simulink model "bandwidth_admittance"  (R2020b)
settings: Solver=ode4  StartTime=0.0  StopTime=5  FixedStep=1e-5  MaxStep=1e-4  RelTol=1e-4  EnableMultiTasking=on
values from neighbouring files (symbols this model uses):
  Be = 2 * sqrt(Ke * Je)    [bandwidth.m]    (also in bandwidth_reference.m = 2 * sqrt(Ke * 0.0001))
  D = 0.1    [bandwidth.m]    (also in bandwidth_reference.m = 0.9; frequency_max_modulation_force.m = 0.9; frequency_max_modulation_force_sea.m = 0.9; frequency_max_modulation_position.m = 0.9)
  dm = 0.0068    [bandwidth.m]    (also in bandwidth_reference.m; frequency_max_modulation_force.m; frequency_max_modulation_force_sea.m; frequency_max_modulation_position.m)
  gear = 103    [bandwidth_reference.m]    (also in frequency_max_position.m; frequency_max_velocity.m; frequency_position.m; frequency_velocity.m)
  Jm = 0.0064    [bandwidth.m]    (also in bandwidth_reference.m = 0.0104; frequency_max_modulation_force.m = 0.0104; frequency_max_modulation_force_sea.m = 0.0104; frequency_max_modulation_position.m = 0.0104)
  Ke = 1e-2    (= 0.01)    [bandwidth.m]    (also in bandwidth_reference.m = 20)
  kt = 1.5038    [bandwidth_reference.m]    (also in frequency_max_modulation_force.m; frequency_max_modulation_force_sea.m; frequency_max_modulation_position.m; frequency_max_modulation_velocity.m)
  P = 15    [bandwidth.m]    (also in bandwidth_reference.m = 1; frequency_max_modulation_force.m = 10; frequency_max_modulation_force_sea.m = 10; frequency_max_modulation_position.m = 10)
  qe = 0    [bandwidth.m]    (also in bandwidth_reference.m)
settings Model: Creator=eldisondimo  LastModifiedBy=filippo
settings DataIOCC: LimitDataPoints=on  SaveOutput=off  SaveTime=off  ReturnWorkspaceOutputs=off
settings OptimizationCC: ExpressionDepthLimit=2147483647  LifeSpan=1
settings DebuggingCC: UnderspecifiedInitializationDetection=Classic  MergeDetectMultiDrivingBlocksExec=none  FcnCallInpInsideContextMsg=warning  AllowSymbolicDim=off  StateNameClashWarn=warning  SFUnexpectedBacktrackingDiag=warning  SFNoUnconditionalDefaultTransitionDiag=warning  SFExecutionAtInitializationDiag=none  ArithmeticOperatorsInVariantConditions=warning
settings SFSimCC: SimUseLocalCustomCode=off  CustomCodeUndefinedFunction=UseInterfaceOnly
settings RTWCC: RTWUseLocalCustomCode=off
settings CodeAppCC: StateflowObjectComments=on
settings GRTTargetCC: TargetLangStandard=C89/C90 (ANSI)  CombineOutputUpdateFcns=off  GRTInterface=on

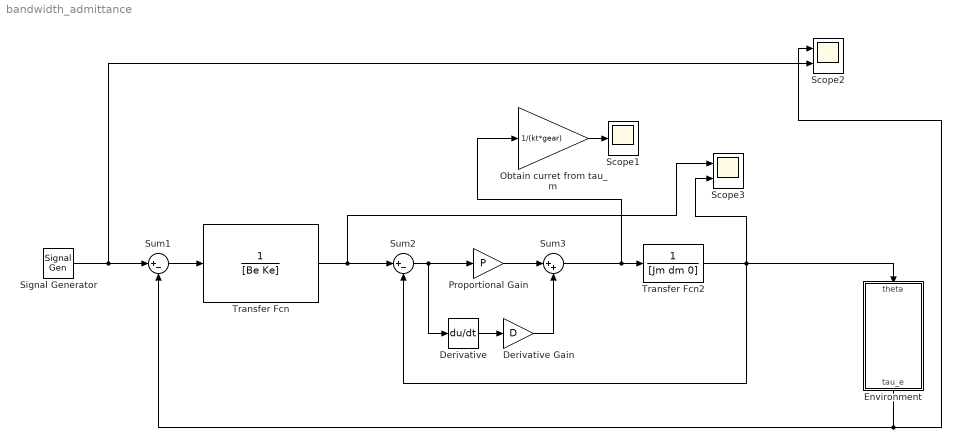
== system bandwidth_admittance ==
  Derivative : Derivative
  Derivative Gain : Gain  Gain=D
  Environment : Subsystem
  Obtain curret from tau_m : Gain  Gain=1/(kt*gear)
  Proportional Gain : Gain  Gain=P
  Scope1 : Scope
  Scope2 : Scope  NumInputPorts=2
  Scope3 : Scope  NumInputPorts=2
  Signal Generator : SignalGenerator  Amplitude=5  Frequency=8  Units=rad/sec
  Sum1 : Sum  Inputs=|+-
  Sum2 : Sum  Inputs=|+-
  Sum3 : Sum  Inputs=|++
  Transfer Fcn : TransferFcn  Denominator=[Be Ke]
  Transfer Fcn2 : TransferFcn  Denominator=[Jm dm 0]
  wires:
  Obtain curret from tau_m/1 -> Scope1/1
  Derivative/1 -> Derivative Gain/1
  Derivative Gain/1 -> Sum3/2
  Proportional Gain/1 -> Sum3/1
  Sum2/1 -> Derivative/1, Proportional Gain/1
  Environment/1(tau_e) -> Sum1/2, Scope2/1
  Sum1/1 -> Transfer Fcn/1
  Sum3/1 -> Transfer Fcn2/1, Obtain curret from tau_m/1
  Transfer Fcn/1 -> Sum2/1, Scope3/1
  Signal Generator/1 -> Sum1/1, Scope2/2
  Transfer Fcn2/1 -> Sum2/2, Scope3/2, Environment/1(theta)

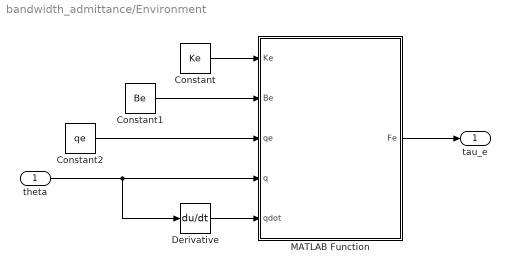
== system bandwidth_admittance/Environment ==
  theta : Inport
  Constant : Constant  Value=Ke
  Constant1 : Constant  Value=Be
  Constant2 : Constant  Value=qe
  Derivative : Derivative
  MATLAB Function : MATLAB Function  TreatAsAtomicUnit=on
  tau_e : Outport  VectorParamsAs1DForOutWhenUnconnected=off
  wires:
  theta/1 -> MATLAB Function/4(q), Derivative/1
  Derivative/1 -> MATLAB Function/5(qdot)
  MATLAB Function/1(Fe) -> tau_e/1
  Constant/1 -> MATLAB Function/1(Ke)
  Constant1/1 -> MATLAB Function/2(Be)
  Constant2/1 -> MATLAB Function/3(qe)

== matlab function bandwidth_admittance/Environment/MATLAB Function ==
  data: Ke input; Be input; qe input; Fe output; q input; qdot input
function Fe = envModel(Ke, Be, qe, q, qdot)
    Fe = Ke * (q - qe) + Be * qdot;
end
